simulink model "sysgenCORDICSinCos_mcode"  (Simulink 7.7)
settings: Solver=ode45  StartTime=0.0  StopTime=500  RelTol=1e-3
undefined symbols (not defined in the file or in its folder): Error_Measurement, sysgenCORDIC_lib
libraries: xbsIndex_r4 x23, dspobslib x9, dspstat3 x4, dspswit3 x2, xbsCopyrightNotice_r4 x1, simulink x1
settings Model: Creator=haibing  LastModifiedBy=douangp
settings DataIOCC: SignalLoggingName=sigsOut
settings OptimizationCC: InlineInvariantSignals=on  InitFltsAndDblsToZero=on
settings DebuggingCC: SaveWithParameterizedLinksMsg=none  SignalResolutionControl=TryResolveAllWithWarning  SolverPrmCheckMsg=none  MultiTaskDSMMsg=warning  MultiTaskCondExecSysMsg=none  StrictBusMsg=None
settings HardwareCC: TargetUnknown=on
settings RTWCC: IncludeERTFirstTime=on
settings GRTTargetCC: TargetFcnLib=ansi_tfl_tmw.mat

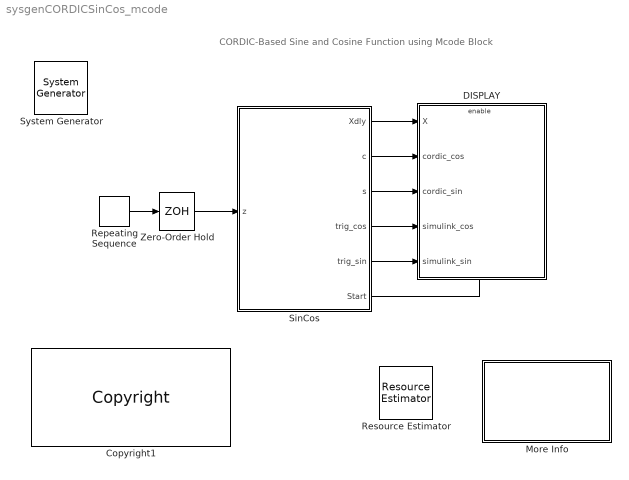
== system sysgenCORDICSinCos_mcode ==
  note: CORDIC-Based Sine and Cosine Function
      | using Mcode Block
  " System Generator" : xbsIndex_r4/ System Generator  Tag=genX  SystemSampleTime=-1  xilinxfamily=kintex7  part=xc7k325t  speed=-1  package=ffg900  synthesis_tool=XST  clock_wrapper=Clock Enables  directory=./sysgenCORDICSinCos_mcode_work  proj_type=Project Navigator  Synth_file=XST Defaults  Impl_file=ISE Defaults  testbench=on  simulink_period=1  sysclk_period=5.1  dcm_input_clock_period=100  incr_netlist=off  trim_vbits=Everywhere in SubSystem  dbl_ovrd=According to Block Masks  core_generation=Not Needed - Already Generated  run_coregen=off  deprecated_control=off  eval_field=0  block_type=sysgen
      settings: block_version=9.2.00
  Copyright1 : xbsCopyrightNotice_r4/Copyright  copyrighttext="Copyright (c) 2011  by  Xilinx, Inc. All rights reserved.<br><br>This file contains proprietary, confidential information of Xilinx, Inc., is distributed under license from Xilinx, Inc., and may be used, copied and/or disclosed only pursuant to the terms of a valid license agreement with Xilinx, Inc. Xilinx hereby grants you a license to use this file solely for design, simulation, implementation and creation of design files limited to Xilinx devices or technologies. Use with non-Xilinx devices or technologies is expressly prohibited and immediately terminates your license unless covered by a separate agreement.<br><br>Xilinx is providing this design, code, or information \"as-is\" solely for use in developing programs and solutions for Xilinx devices, with no obligation on the part of Xilinx to provide support. By providing this design, code, or information as one possible implementation of this feature, application or standard, Xilinx is making no representation that this implementation is free from any claims of infringement. You are responsible for obtaining any rights you may require for your implementation. Xilinx expressly disclaims any warranty whatsoever with respect to the adequacy of the implementation, including but not limited to any warranties or representations that this implementation is free from claims of infringement, implied warranties of merchantability or fitness for a particular purpose.<br><br>Xilinx products are not intended for use in life support appliances, devices, or systems. Use in such applications is expressly prohibited.<br><br>Any modifications that are made to the Source Code are done at the user's sole risk and will be unsupported.<br><br>This copyright and support notice must be retained as part of this text at all times. (c) Copyright 1995-2011 Xilinx, Inc. All rights reserved."  block_type=copyright
      settings: block_version=10.1.00
      settings: infoedit=|
      | Copyright(C) 2008 by  Xilinx, Inc. All rights reserved.<br>
      | <br>
      | This file contains proprietary, confidential information of Xilinx, Inc., is distributed under license
      | from Xilinx, Inc., and may be used, copied and/or disclosed only pursuant to the terms of a valid license
      | agreement with Xilinx, Inc. Xilinx hereby grants you a license to use this file solely for design,
      | simulation, implementation and creation of design files limited to Xilinx devices or technologies. Use
      | with non-Xilinx devices or technologies is expressly prohibited and immediately terminates your license
      | unless covered by a separate agreement.<br>
      | <br>
      | Xilinx is providing this design, code, or information "as-is" solely for use in developing programs and
      | solutions for Xilinx devices, with no obligation on the part of Xilinx to provide support. By providing
      | this design, code, or information as one possible implementation of this feature, application or standard,
      | Xilinx is making no representation that this implementation is free from any claims of infringement. You
      | are responsible for obtaining any rights you may require for your implementation. Xilinx expressly disclaims
      | any warranty whatsoever with respect to the adequacy of the implementation, including but not limited to any
      | warranties or representations that this implementation is free from claims of infringement, implied warranties
      | of merchantability or fitness for a particular purpose.<br>
      | <br>
      | Xilinx products are not intended for use in life support appliances, devices, or systems. Use in such
      | applications is expressly prohibited.<br>
      | <br>
      | Any modifications that are made to the Source Code are done at the user's sole risk and will be unsupported.<br>
      | <br>
      | This copyright and support notice must be retained as part of this text at all times.
      | (c) Copyright 1995-2008 Xilinx, Inc. All rights reserved.
  DISPLAY : Subsystem  TreatAsAtomicUnit=on
  More Info : Subsystem
      mask Display: disp('Double click\n for\n more information.')
  Repeating Sequence : simulink/Sources/Repeating Sequence  SystemSampleTime=-1  rep_seq_t=0:1:201  rep_seq_y=-pi:1/32:pi
  Resource Estimator : xbsIndex_r4/Resource Estimator  Tag=resEstTag  Slices=324  FFs=532  BRAMs=0  LUTs=556  IOBs=48  EBMs=0  TBUFs=0  xl_use_estimator_area=off  est_options=Estimate  xl_estimator_area=[324 532 0 556 48 0 0]  mrp_directory=./sysgenCORDIC_work_test  simulink_period=1  block_type=resource_estimator
      settings: AttributesFormatString=Resource\nEstimator  block_version=9.2.00
  SinCos : Subsystem  mask{pe_stages=8, pe_nbits=16, pe_binpt=13}
      mask prompts: pe_stages "Stages"; pe_nbits "Data Width"; pe_binpt "Binary Point"
      mask init:
      | [bg,fg] = xlcmap('XBlock',0);
      | iPos = get_param(gcb,'Position');
      | iWidth=iPos(3)-iPos(1); iHeight=iPos(4)-iPos(2);
      | iCx=iWidth/2;
      | iCy=iHeight/2;
      | [logoX, logoY] = xlogo(iPos);
      | 
      | pipeline = ones(1, pe_stages);
      | 
      | stages = round(sum(abs(pe_stages)));
      | if (stages == 0)
      | 	stages = 1;
      | end
      | x = zeros(1,stages);
      | pipe_size = max(size(pipeline));
      | if pipe_size >= stages
      | 	x(1,1:stages) = pipeline(1,1:stages);
      | else
      | 	x(1,1:pipe_size) = pipeline(1,1:pipe_size);
      | end
      | 
      | cordic_pe = find_system(gcb, 'LookUnderMasks', 'all', 'FollowLinks','on','masktype', 'CORDIC parallel PE');
      | a = find_system(cordic_pe{1}, 'LookUnderMasks', 'all', 'FollowLinks','on','masktype', 'CORDIC iteration PE');
      | prev_stages = length(a);
      | 
      | find_system(bdroot(gcs), 'lookUnderMasks', 'all', 'FollowLinks','on');
      | 
      | if (stages ~=prev_stages)
      |   pipeline=x;
      |     
      |   for i= 2:length(a)
      |     for j=1:3
      | 	  delete_line(cordic_pe{1}, ['CORDIC PE' int2str(i-1) '/' int2str(j)], ['CORDIC PE' int2str(i) '/' int2str(j)]);
      |     end
      |   end
      |     if length(a)>0,
      |       delete_line(cordic_pe{1}, 'x/1', 'CORDIC PE1/1');
      |       delete_line(cordic_pe{1}, 'y/1', 'CORDIC PE1/2');
      |       delete_line(cordic_pe{1}, 'z/1', 'CORDIC PE1/3');
      |       delete_line(cordic_pe{1}, ['CORDIC PE' int2str(length(a)) '/1'],'X/1');
      |       delete_line(cordic_pe{1}, ['CORDIC PE' int2str(length(a)) '/2'],'Y/1');
      |       delete_line(cordic_pe{1}, ['CORDIC PE' int2str(length(a)) '/3'],'Terminator/1');
      |     elseif length(a)==0
      |       temp_port=get_param([cordic_pe{1} '/x'],'porthandles');
      |       temp_line=get_param(temp_port.Outport,'line');
      |       if temp_line>=0  delete_line(temp_line); end
      |       temp_port=get_param([cordic_pe{1} '/y'],'porthandles');
      |       temp_line=get_param(temp_port.Outport,'line');
      |       if temp_line>=0  delete_line(temp_line); end
      |       temp_port=get_param([cordic_pe{1} '/z'],'porthandles');
      |       temp_line=get_param(temp_port.Outport,'line');
      |       if temp_line>=0  delete_line(temp_line); end
      |     end
      | 
      |     for i=2:length(a)
      |       delete_block(a{i});
      |     end
      |     for i=2:stages,
      |         add_block([cordic_pe{1} '/CORDIC PE1'], [cordic_pe{1} '/CORDIC PE' int2str(i)], 'ii', int2str(i-1),'pe_nbits', 'pe_nbits','pe_binpt', 'pe_binpt','pipeline',['pipeline(1,' int2str(i) ')'],'position',[150+(i-1)*125, 70, 205+(i-1)*125, 130]);
      |     end
      | 
      |     for i= 2:stages,
      |       for j=1:3
      | 		add_line(cordic_pe{1}, ['CORDIC PE' int2str(i-1) '/' int2str(j)], ['CORDIC PE' int2str(i) '/' int2str(j)], 'autorouting', 'on');
      |       end
      |     end
      | 
      |     if stages==0
      |       add_line(cordic_pe{1}, 'x/1', 'X/1', 'autorouting', 'on');
      |       add_line(cordic_pe{1}, 'y/1', 'Terminator/1', 'autorouting', 'on');
      |       add_line(cordic_pe{1}, 'z/1', 'Z/1', 'autorouting', 'on');
      |     elseif stages>0
      |       add_line(cordic_pe{1}, 'x/1', 'CORDIC PE1/1', 'autorouting', 'on');
      |       add_line(cordic_pe{1}, 'y/1', 'CORDIC PE1/2', 'autorouting', 'on');
      |       add_line(cordic_pe{1}, 'z/1', 'CORDIC PE1/3', 'autorouting', 'on');
      | 
      |       set_param([cordic_pe{1} '/' 'X'], 'Position', [150+stages*125, 72, 180+stages*125, 86]);
      |       set_param([cordic_pe{1} '/' 'Y'], 'Position', [210+stages*125, 92, 225+stages*125, 108]);
      |       set_param([cordic_pe{1} '/' 'Terminator'], 'Position', [240+stages*125, 113, 270+stages*125, 127]);
      | 
      |       add_line(cordic_pe{1}, ['CORDIC PE' int2str(stages) '/1'], 'X/1', 'autorouting', 'on');
      |       add_line(cordic_pe{1}, ['CORDIC PE' int2str(stages) '/2'], 'Y/1', 'autorouting', 'on');
      |       add_line(cordic_pe{1}, ['CORDIC PE' int2str(stages) '/3'],'Terminator/1', 'autorouting', 'on');
      | 
      |       % force a "compile" of the constituent constant blocks to
      |       % workaround a data propagation problem
      |       find_system(cordic_pe{1}, 'LookUnderMasks', 'all', 'FollowLinks', 'on', 'MaskType','Xilinx Constant Block');
      |   end
      | end
      | latency = sum(x) + 5;
      | str = sprintf('-%d',latency);
      mask Display:
      | patch([0 iWidth iWidth 0],[0 0 iHeight iHeight] , bg);
      | patch(logoX,logoY , fg);
      | 
      | text(iCx-6,iCy,'z');
      | text(iCx,iCy+4,str);
      | 
      | port_label('input',1,'z');
      | port_label('output',1,'z_dly');
      | port_label('output',2,'cordic_cos');
      | port_label('output',3,'cordic_sin');
      | port_label('output',4,'simulink_cos');
      | port_label('output',5,'simulink_sin');
      | port_label('output',6,'Start');
      | plot([0 0 iWidth iWidth 0], [0 iHeight iHeight 0 0]);
  Zero-Order Hold : ZeroOrderHold
  wires:
  Repeating Sequence/1 -> Zero-Order Hold/1
  Zero-Order Hold/1 -> SinCos/1(z)
  SinCos/1(Xdly) -> DISPLAY/1(X)
  SinCos/2(c) -> DISPLAY/2(cordic_cos)
  SinCos/3(s) -> DISPLAY/3(cordic_sin)
  SinCos/4(trig_cos) -> DISPLAY/4(simulink_cos)
  SinCos/5(trig_sin) -> DISPLAY/5(simulink_sin)
  SinCos/6(Start) -> DISPLAY/Enable

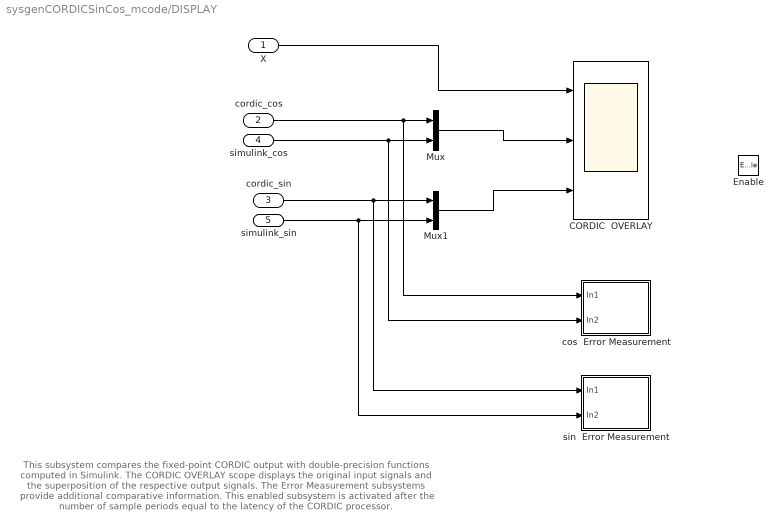
== system sysgenCORDICSinCos_mcode/DISPLAY ==
  note: This subsystem compares the fixed-point CORDIC output with double-precision functions computed in Simulink. The CORDIC OVERLAY scope
      | displays the original input signals and the superposition of the respective output signals.  The Error Measurement subsystems provide additional
      | comparative information.  This enabled subsystem is activated after the number of sample periods equal to the latency of the CORDIC processor.
  X : Inport
  cordic_cos : Inport  Port=2
  cordic_sin : Inport  Port=3
  simulink_cos : Inport  Port=4
  simulink_sin : Inport  Port=5
  Enable : EnablePort
  CORDIC  OVERLAY : Scope  NumInputPorts=3
      settings: TimeRange=500  YMin=-4~-1~-1.5  YMax=4~1.5~1.5
  Mux : Mux  Inputs=2
  Mux1 : Mux  Inputs=2
  cos  Error Measurement : Subsystem  AncestorBlock=sysgenCORDIC_lib/Error_Measurement
      mask Type: Error Measurement
  sin  Error Measurement : Subsystem
      mask Type: Error Measurement
  wires:
  Mux/1 -> CORDIC  OVERLAY/2
  Mux1/1 -> CORDIC  OVERLAY/3
  simulink_sin/1 -> sin  Error Measurement/2(In2), Mux1/2
  cordic_sin/1 -> sin  Error Measurement/1(In1), Mux1/1
  X/1 -> CORDIC  OVERLAY/1
  simulink_cos/1 -> cos  Error Measurement/2(In2), Mux/2
  cordic_cos/1 -> cos  Error Measurement/1(In1), Mux/1

== system sysgenCORDICSinCos_mcode/More Info ==
  note: CORDIC-Based Sine and Cosine Function using Mcode Block
  note: This design implements a fully parallel CORDIC  (COordinate Rotation DIgital Computer) algorithm in rotational mode that computes
      | the sine and cosine of the input angle z between +/- pi.
      |
      | The CORDIC algorithm is attractive for an FPGA implementation because it consists primarily of shift and add operations.
      | An N-bit adder/subtractor  requiries only N/2 logic slices.  The CORDIC subsystem is masked, and allows customization of bit precision,
      | the number of processing elements (PEs) in the CORDIC engine and the ability to pieline each individual stage.
      |
      |
      | References:
      | J. E. Volder, "The CORDIC Trigonometric Computing Technique", IRE Trans. On Electronic Computers, Vol. EC-8,  1959, pp. 330-334.
      | J. S. Walther, "A Unified Algorithm for Elementary Functions", Spring Joint Computer Conference (1971) pp. 379-385.
      | Yu Hen Hu, "CORDIC-Based VLSI Architectures for Digital Signal Processing", IEEE Signal Processing Magazine, pp. 17-34, July 1992.

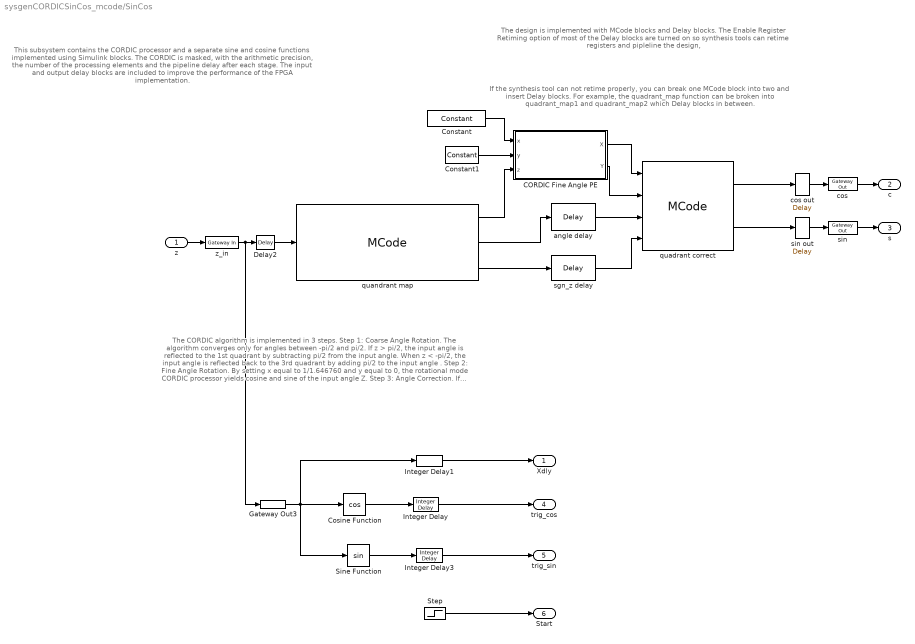
== system sysgenCORDICSinCos_mcode/SinCos ==
  note: This subsystem contains the CORDIC processor and a separate sine and cosine functions implemented using Simulink blocks.
      | The CORDIC is masked, with the arithmetic precision, the number of the processing elements and the pipeline delay after each
      | stage. The input and output delay blocks are included to improve the performance of the FPGA implementation.
  note: The CORDIC algorithm is implemented in 3 steps.
      |
      | Step 1: Coarse Angle Rotation.  The algorithm converges only for angles between -pi/2 and pi/2. If  z > pi/2, the input angle is reflected
      |  to the 1st quadrant by subtracting pi/2 from the input angle. When z < -pi/2, the input angle is reflected back to the 3rd quadrant by adding
      | pi/2 to the input angle .
      |
      | Step 2: Fine Angle Rotation.  By setting x equal to 1/1.646760 and y equal to 0, the rotational mode CORDIC processor yields cosine and sine
      | of the input angle Z.
      |
      | Step 3: Angle Correction. If there was a reflection applied in Step 1, this step applies the appropriate correction .
  note: If the synthesis tool can not retime properly, you can break one
      | MCode block into two and insert Delay blocks. For example,
      | the quadrant_map function can be broken into quadrant_map1
      | and quadrant_map2 which Delay blocks in between.
  note: The design is implemented with MCode blocks and Delay blocks.
      | The Enable Register Retiming option of most of the Delay blocks
      | are turned on so synthesis tools can retime registers and
      | pipleline the design,
  z : Inport
  CORDIC Fine Angle PE : Subsystem  mask(CORDIC parallel PE){}
      mask init:
      | [bg,fg] = xlcmap('XBlock',0);
      | iPos = get_param(gcb,'Position');
      | iWidth=iPos(3)-iPos(1); iHeight=iPos(4)-iPos(2);
      | iCx=iWidth/2;
      | iCy=iHeight/2;
      | [logoX, logoY] = xlogo(iPos);
      mask Display:
      | patch([0 iWidth iWidth 0],[0 0 iHeight iHeight] , bg);
      | patch(logoX,logoY , fg);
      | port_label('input',1,'x');
      | port_label('input',2,'y');
      | port_label('input',3,'z');
      | port_label('output',1,'X');
      | port_label('output',2,'Y');
      | plot([0 0 iWidth iWidth 0], [0 iHeight iHeight 0 0]);
  Constant : xbsIndex_r4/Constant  const=1/1.646760  gui_display_data_type=Fixed-point  arith_type=Unsigned  n_bits=pe_nbits  bin_pt=pe_binpt  preci_type=Single  exp_width=8  frac_width=24  explicit_period=on  period=1  equ=P=C  opselect=C  inp2=PCIN>>17  opr=+  inp1=P  carry=CIN  dbl_ovrd=off  block_type=constant
      settings: block_version=VER_STRING_GOES_HERE
  Constant1 : xbsIndex_r4/Constant  const=0  gui_display_data_type=Fixed-point  arith_type=Unsigned  n_bits=pe_nbits  bin_pt=pe_binpt  preci_type=Single  exp_width=8  frac_width=24  explicit_period=on  period=1  equ=P=C  opselect=C  inp2=PCIN>>17  opr=+  inp1=P  carry=CIN  dbl_ovrd=off  block_type=constant
      settings: block_version=VER_STRING_GOES_HERE
  Cosine Function : Trigonometry  Operator=cos
  Delay2 : xbsIndex_r4/Delay  rst=off  infoeditControl=Selection of Reset will increase slice count due to use of real FFs and instead of SRLs  en=off  latency=1  dbl_ovrd=off  reg_retiming=off  block_type=delay
      settings: infoedit="Delay line having  configurable length.<P><P>Hardware notes: A delay line is a chain, each link of which is an SRL16 followed by a flip-flop. If register retiming is enabled, the delay line is a chain of flip-flops."  xl_area=[8 16 0 0 0 0 0]  block_version=VER_STRING_GOES_HERE
  Gateway Out3 : xbsIndex_r4/Gateway Out  hdl_port=off  timing_constraint=None  locs_specified=off  LOCs={}  block_type=gatewayout
      settings: infoedit="Gateway out block.  Converts Xilinx fixed point inputs into ouputs of type Simulink integer, double, or fixed point.<P><P>Hardware notes:  In hardware these blocks become top level output ports or are discarded, depending on how they are configured."  xl_area=[0 0 0 0 0 0 0]  block_version=VER_STRING_GOES_HERE
  Integer Delay : dspobslib/Integer Delay  delay=latency  ic=0  reset_popup=None
  Integer Delay1 : dspobslib/Integer Delay  delay=latency  ic=0  reset_popup=None
  Integer Delay3 : dspobslib/Integer Delay  delay=latency  ic=0  reset_popup=None
  Sine Function : Trigonometry
  Step : Step  Time=latency  SampleTime=1
  angle delay : xbsIndex_r4/Delay  rst=off  infoeditControl=Selection of Reset will increase slice count due to use of real FFs and instead of SRLs  en=off  latency=sum(pipeline)  dbl_ovrd=off  reg_retiming=off  block_type=delay
      settings: infoedit="Delay line having  configurable length.<P><P>Hardware notes: A delay line is a chain, each link of which is an SRL16 followed by a flip-flop. If register retiming is enabled, the delay line is a chain of flip-flops."  xl_area=[0, 0, 0, 0, 0, 0, 0]  block_version=VER_STRING_GOES_HERE
  cos : xbsIndex_r4/Gateway Out  hdl_port=on  timing_constraint="Data Rate;  Set 'FAST' Attribute"  locs_specified=off  LOCs={}  block_type=gatewayout
      settings: infoedit="Gateway out block.  Converts Xilinx fixed point inputs into ouputs of type Simulink integer, double, or fixed point.<P><P>Hardware notes:  In hardware these blocks become top level output ports or are discarded, depending on how they are configured."  xl_area=[0 0 0 0 16 0 0]  block_version=VER_STRING_GOES_HERE
  cos out : xbsIndex_r4/Delay  rst=off  infoeditControl=Selection of Reset will increase slice count due to use of real FFs and instead of SRLs  en=off  latency=1  dbl_ovrd=off  reg_retiming=off  block_type=delay
      settings: infoedit="Delay line having  configurable length.<P><P>Hardware notes: A delay line is a chain, each link of which is an SRL16 followed by a flip-flop. If register retiming is enabled, the delay line is a chain of flip-flops."  xl_area=[0, 0, 0, 0, 0, 0, 0]  block_version=VER_STRING_GOES_HERE
  quadrant correct : xbsIndex_r4/MCode  mfname=quadrant_correct_lat  explicit_period=off  period=1  dbl_ovrd=off  enable_stdout=off  enable_debug=off  suppress_output=off  defparams={'nbits', pe_nbits,'binpt', pe_binpt,'lat',1}  hide_port_list={}  block_type=mcode
      settings: xl_area=[0, 0, 0, 0, 0, 0, 0]  block_version=8.1
  quandrant map : xbsIndex_r4/MCode  mfname=quadrant_map_lat2  explicit_period=off  period=1  dbl_ovrd=off  enable_stdout=off  enable_debug=off  suppress_output=off  defparams={'nbits', pe_nbits,'binpt', pe_binpt,'lat',2}  hide_port_list={}  block_type=mcode
      settings: xl_area=[0, 0, 0, 0, 0, 0, 0]  block_version=8.1
  sgn_z delay : xbsIndex_r4/Delay  rst=off  infoeditControl=Selection of Reset will increase slice count due to use of real FFs and instead of SRLs  en=off  latency=sum(pipeline)  dbl_ovrd=off  reg_retiming=off  block_type=delay
      settings: infoedit="Delay line having  configurable length.<P><P>Hardware notes: A delay line is a chain, each link of which is an SRL16 followed by a flip-flop. If register retiming is enabled, the delay line is a chain of flip-flops."  xl_area=[0, 0, 0, 0, 0, 0, 0]  block_version=VER_STRING_GOES_HERE
  sin : xbsIndex_r4/Gateway Out  hdl_port=on  timing_constraint="Data Rate;  Set 'FAST' Attribute"  locs_specified=off  LOCs={}  block_type=gatewayout
      settings: infoedit="Gateway out block.  Converts Xilinx fixed point inputs into ouputs of type Simulink integer, double, or fixed point.<P><P>Hardware notes:  In hardware these blocks become top level output ports or are discarded, depending on how they are configured."  xl_area=[0 0 0 0 16 0 0]  block_version=VER_STRING_GOES_HERE
  sin out : xbsIndex_r4/Delay  rst=off  infoeditControl=Selection of Reset will increase slice count due to use of real FFs and instead of SRLs  en=off  latency=1  dbl_ovrd=off  reg_retiming=off  block_type=delay
      settings: infoedit="Delay line having  configurable length.<P><P>Hardware notes: A delay line is a chain, each link of which is an SRL16 followed by a flip-flop. If register retiming is enabled, the delay line is a chain of flip-flops."  xl_area=[0, 0, 0, 0, 0, 0, 0]  block_version=VER_STRING_GOES_HERE
  z_in : xbsIndex_r4/Gateway In  gui_display_data_type=Fixed-point  arith_type="Signed  (2's comp)"  n_bits=pe_nbits  bin_pt=pe_binpt  preci_type=Single  exp_width=8  frac_width=24  quantization="Round  (unbiased: +/- Inf)"  overflow=Saturate  period=1  dbl_ovrd=off  timing_constraint=None  locs_specified=off  LOCs={}  hdl_port=on  block_type=gatewayin
      settings: infoedit="Gateway in block.  Converts inputs of type Simulink integer, double and fixed point to  Xilinx fixed point type.<P><P>Hardware notes:  In hardware these blocks become top level input ports."  xl_area=[0 0 0 0 16 0 0]  block_version=VER_STRING_GOES_HERE
  Xdly : Outport
  c : Outport  Port=2
  s : Outport  Port=3
  trig_cos : Outport  Port=4
  trig_sin : Outport  Port=5
  Start : Outport  Port=6
  wires:
  z_in/1 -> Delay2/1, Gateway Out3/1
  quandrant map/1 -> CORDIC Fine Angle PE/3(z)
  CORDIC Fine Angle PE/1(X) -> quadrant correct/1
  CORDIC Fine Angle PE/2(Y) -> quadrant correct/2
  angle delay/1 -> quadrant correct/3
  sgn_z delay/1 -> quadrant correct/4
  Constant/1 -> CORDIC Fine Angle PE/1(x)
  Constant1/1 -> CORDIC Fine Angle PE/2(y)
  Delay2/1 -> quandrant map/1
  z/1 -> z_in/1
  cos out/1 -> cos/1
  sin out/1 -> sin/1
  Gateway Out3/1 -> Integer Delay1/1, Sine Function/1, Cosine Function/1
  Step/1 -> Start/1
  Integer Delay3/1 -> trig_sin/1
  Integer Delay/1 -> trig_cos/1
  Sine Function/1 -> Integer Delay3/1
  Integer Delay1/1 -> Xdly/1
  Cosine Function/1 -> Integer Delay/1
  cos/1 -> c/1
  sin/1 -> s/1
  quandrant map/2 -> angle delay/1
  quandrant map/3 -> sgn_z delay/1
  quadrant correct/1 -> cos out/1
  quadrant correct/2 -> sin out/1

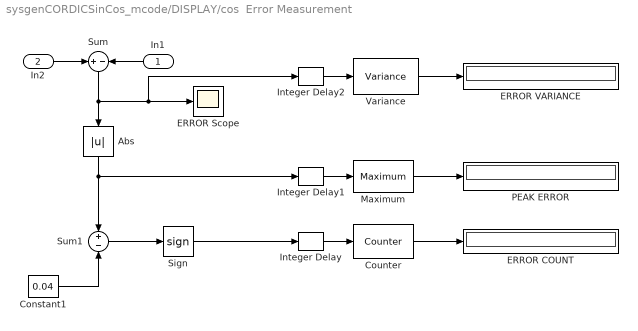
== system sysgenCORDICSinCos_mcode/DISPLAY/cos  Error Measurement ==
  In1 : Inport
  In2 : Inport  Port=2
  Abs : Abs  SaturateOnIntegerOverflow=on
  Constant1 : Constant  Value=0.04
  Counter : dspswit3/Counter  Direction=Up  CountEvent=Rising edge  CounterSize=User defined  MaxCount=200000000  InitialCount=0  Output=Count  HitValue=32  ResetInput=off  SamplesPerFrame=1  Ts=1  CntDtype=double  HitDtype=Logical
  ERROR Scope : Scope
      settings: TimeRange=10000  YMin=-0.0006  YMax=0.0005  SaveName=ScopeData2
  ERROR COUNT : Display
      settings: Format=long_e
  ERROR VARIANCE : Display
      settings: Format=long_e
  Integer Delay : dspobslib/Integer Delay  delay=1  ic=0  reset_popup=None
  Integer Delay1 : dspobslib/Integer Delay  delay=1  ic=0  reset_popup=None
  Integer Delay2 : dspobslib/Integer Delay  delay=1  ic=0  reset_popup=None
  Maximum : dspstat3/Maximum  fcn=Running  reset=None  InputProcessing=Inherited (this choice will be removed - see release notes)  indexBase=One  operateOver=Each column  Dimension=1  colComp=on  operation=maximum  roiEnable=off  roiType=Rectangles  roiPortion=Entire ROI  roiOutput=Individual statistics for each ROI  roiFlag=off  accumDataTypeStr=Inherit: Same as product output  accumLastDataTypeStr=Inherit: Same as product output  roundingMode=Floor  overflowMode=off
  PEAK ERROR : Display
      settings: Format=long_e
  Sign : Signum
  Sum : Sum  Inputs=+-  SaturateOnIntegerOverflow=on  InputSameDT=on  OutDataTypeStr=Inherit: Same as first input
  Sum1 : Sum  Inputs=+-  SaturateOnIntegerOverflow=on  InputSameDT=on  OutDataTypeStr=Inherit: Same as first input
  Variance : dspstat3/Variance  run=on  reset_popup=None  InputProcessing=Inherited (this choice will be removed - see release notes)  directionMode=Each column  dimension=1  treatSBRowAsCol=on  roiEnable=off  roiType=Rectangles  roiPortion=Entire ROI  roiOutput=Individual statistics for each ROI  roiFlag=off  roundingMode=Floor  overflowMode=off
  wires:
  In2/1 -> Sum/1
  In1/1 -> Sum/2
  Integer Delay2/1 -> Variance/1
  Integer Delay1/1 -> Maximum/1
  Integer Delay/1 -> Counter/1
  Maximum/1 -> PEAK ERROR/1
  Variance/1 -> ERROR VARIANCE/1
  Counter/1 -> ERROR COUNT/1
  Sign/1 -> Integer Delay/1
  Sum1/1 -> Sign/1
  Abs/1 -> Integer Delay1/1, Sum1/1
  Constant1/1 -> Sum1/2
  Sum/1 -> Integer Delay2/1, ERROR Scope/1, Abs/1

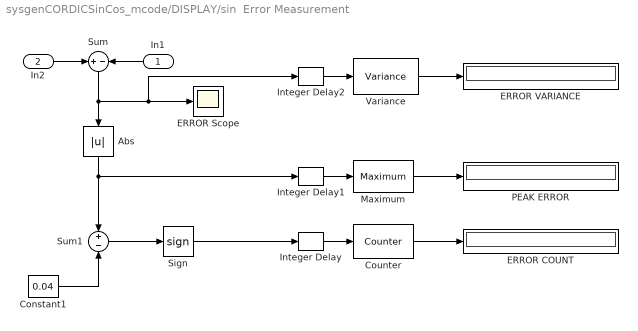
== system sysgenCORDICSinCos_mcode/DISPLAY/sin  Error Measurement ==
  In1 : Inport
  In2 : Inport  Port=2
  Abs : Abs  SaturateOnIntegerOverflow=on
  Constant1 : Constant  Value=0.04
  Counter : dspswit3/Counter  Direction=Up  CountEvent=Rising edge  CounterSize=User defined  MaxCount=200000000  InitialCount=0  Output=Count  HitValue=32  ResetInput=off  SamplesPerFrame=1  Ts=1  CntDtype=double  HitDtype=Logical
  ERROR Scope : Scope
      settings: TimeRange=10000  YMin=-0.0006  YMax=0.0005  SaveName=ScopeData2
  ERROR COUNT : Display
      settings: Format=long_e
  ERROR VARIANCE : Display
      settings: Format=long_e
  Integer Delay : dspobslib/Integer Delay  delay=1  ic=0  reset_popup=None
  Integer Delay1 : dspobslib/Integer Delay  delay=1  ic=0  reset_popup=None
  Integer Delay2 : dspobslib/Integer Delay  delay=1  ic=0  reset_popup=None
  Maximum : dspstat3/Maximum  fcn=Running  reset=None  InputProcessing=Inherited (this choice will be removed - see release notes)  indexBase=One  operateOver=Each column  Dimension=1  colComp=on  operation=maximum  roiEnable=off  roiType=Rectangles  roiPortion=Entire ROI  roiOutput=Individual statistics for each ROI  roiFlag=off  accumDataTypeStr=Inherit: Same as product output  accumLastDataTypeStr=Inherit: Same as product output  roundingMode=Floor  overflowMode=off
  PEAK ERROR : Display
      settings: Format=long_e
  Sign : Signum
  Sum : Sum  Inputs=+-  SaturateOnIntegerOverflow=on  InputSameDT=on  OutDataTypeStr=Inherit: Same as first input
  Sum1 : Sum  Inputs=+-  SaturateOnIntegerOverflow=on  InputSameDT=on  OutDataTypeStr=Inherit: Same as first input
  Variance : dspstat3/Variance  run=on  reset_popup=None  InputProcessing=Inherited (this choice will be removed - see release notes)  directionMode=Each column  dimension=1  treatSBRowAsCol=on  roiEnable=off  roiType=Rectangles  roiPortion=Entire ROI  roiOutput=Individual statistics for each ROI  roiFlag=off  roundingMode=Floor  overflowMode=off
  wires:
  In2/1 -> Sum/1
  In1/1 -> Sum/2
  Integer Delay2/1 -> Variance/1
  Integer Delay1/1 -> Maximum/1
  Integer Delay/1 -> Counter/1
  Maximum/1 -> PEAK ERROR/1
  Variance/1 -> ERROR VARIANCE/1
  Counter/1 -> ERROR COUNT/1
  Sign/1 -> Integer Delay/1
  Sum1/1 -> Sign/1
  Abs/1 -> Integer Delay1/1, Sum1/1
  Constant1/1 -> Sum1/2
  Sum/1 -> Integer Delay2/1, ERROR Scope/1, Abs/1

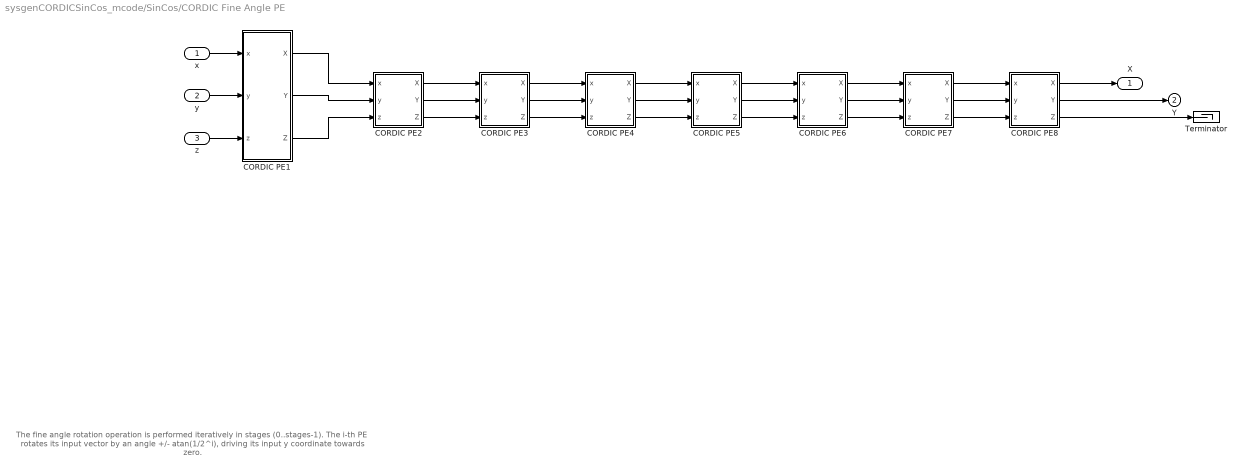
== system sysgenCORDICSinCos_mcode/SinCos/CORDIC Fine Angle PE ==
  note: The fine angle rotation operation is performed iteratively in stages (0..stages-1).
      | The i-th PE rotates its input vector by an angle +/- atan(1/2^i), driving its input y coordinate towards zero.
  x : Inport
  y : Inport  Port=2
  z : Inport  Port=3
  CORDIC PE1 : Subsystem  mask(CORDIC iteration PE){ii=0, pe_nbits=pe_nbits, pe_binpt=pe_binpt, epsilon_k_fcn=atan, epsilon_k=, pipeline=pipeline(1,1)}
      mask prompts: ii "Iteration Index ii"; pe_nbits "Number of X,Y,Z Bits"; pe_binpt "X,Y,Z Binary Point Position"; epsilon_k_fcn "Epsilon_k Function"; pipeline "Pipeline Latency"
      mask init:
      | [bg,fg] = xlcmap('XBlock',0);
      | iPos = get_param(gcb,'Position');
      | iWidth=iPos(3)-iPos(1); iHeight=iPos(4)-iPos(2);
      | iCx=iWidth/2;
      | iCy=iHeight/2;
      | [logoX, logoY] = xlogo(iPos);
      | 
      | set_param(gcb, 'LinkStatus', 'none');
      | switch epsilon_k_fcn
      |   case 1
      |     epsilon_k = atan(1/2^ii);
      |   case 2
      |     epsilon_k = atanh(1/2^ii);
      | end
      mask StyleString: edit,edit,edit,popup(atan|atanh),edit,edit
      mask Display:
      | patch([0 iWidth iWidth 0],[0 0 iHeight iHeight] , bg);
      | patch(logoX,logoY , fg);
      | port_label('input',1,'x');
      | port_label('input',2,'y');
      | port_label('input',3,'z');
      | 
      | port_label('output',1,'X');
      | port_label('output',2,'Y');
      | port_label('output',3,'Z');
      | plot([0 0 iWidth iWidth 0], [0 iHeight iHeight 0 0]);
  CORDIC PE2 : Subsystem  mask(CORDIC iteration PE){ii=1, pe_nbits=pe_nbits, pe_binpt=pe_binpt, epsilon_k_fcn=atan, epsilon_k=, pipeline=pipeline(1,2)}
      mask prompts: ii "Iteration Index ii"; pe_nbits "Number of X,Y,Z Bits"; pe_binpt "X,Y,Z Binary Point Position"; epsilon_k_fcn "Epsilon_k Function"; pipeline "Pipeline Latency"
      mask init: same as sysgenCORDICSinCos_mcode/SinCos/CORDIC Fine Angle PE/CORDIC PE1
      mask StyleString: edit,edit,edit,popup(atan|atanh),edit,edit
      mask Display:
      | patch([0 iWidth iWidth 0],[0 0 iHeight iHeight] , bg);
      | patch(logoX,logoY , fg);
      | port_label('input',1,'x');
      | port_label('input',2,'y');
      | port_label('input',3,'z');
      | 
      | port_label('output',1,'X');
      | port_label('output',2,'Y');
      | port_label('output',3,'Z');
      | plot([0 0 iWidth iWidth 0], [0 iHeight iHeight 0 0]);
  CORDIC PE3 : Subsystem  mask(CORDIC iteration PE){ii=2, pe_nbits=pe_nbits, pe_binpt=pe_binpt, epsilon_k_fcn=atan, epsilon_k=, pipeline=pipeline(1,3)}
      mask prompts: ii "Iteration Index ii"; pe_nbits "Number of X,Y,Z Bits"; pe_binpt "X,Y,Z Binary Point Position"; epsilon_k_fcn "Epsilon_k Function"; pipeline "Pipeline Latency"
      mask init: same as sysgenCORDICSinCos_mcode/SinCos/CORDIC Fine Angle PE/CORDIC PE1
      mask StyleString: edit,edit,edit,popup(atan|atanh),edit,edit
      mask Display:
      | patch([0 iWidth iWidth 0],[0 0 iHeight iHeight] , bg);
      | patch(logoX,logoY , fg);
      | port_label('input',1,'x');
      | port_label('input',2,'y');
      | port_label('input',3,'z');
      | 
      | port_label('output',1,'X');
      | port_label('output',2,'Y');
      | port_label('output',3,'Z');
      | plot([0 0 iWidth iWidth 0], [0 iHeight iHeight 0 0]);
  CORDIC PE4 : Subsystem  mask(CORDIC iteration PE){ii=3, pe_nbits=pe_nbits, pe_binpt=pe_binpt, epsilon_k_fcn=atan, epsilon_k=, pipeline=pipeline(1,4)}
      mask prompts: ii "Iteration Index ii"; pe_nbits "Number of X,Y,Z Bits"; pe_binpt "X,Y,Z Binary Point Position"; epsilon_k_fcn "Epsilon_k Function"; pipeline "Pipeline Latency"
      mask init: same as sysgenCORDICSinCos_mcode/SinCos/CORDIC Fine Angle PE/CORDIC PE1
      mask StyleString: edit,edit,edit,popup(atan|atanh),edit,edit
      mask Display:
      | patch([0 iWidth iWidth 0],[0 0 iHeight iHeight] , bg);
      | patch(logoX,logoY , fg);
      | port_label('input',1,'x');
      | port_label('input',2,'y');
      | port_label('input',3,'z');
      | 
      | port_label('output',1,'X');
      | port_label('output',2,'Y');
      | port_label('output',3,'Z');
      | plot([0 0 iWidth iWidth 0], [0 iHeight iHeight 0 0]);
  CORDIC PE5 : Subsystem  mask(CORDIC iteration PE){ii=4, pe_nbits=pe_nbits, pe_binpt=pe_binpt, epsilon_k_fcn=atan, epsilon_k=, pipeline=pipeline(1,5)}
      mask prompts: ii "Iteration Index ii"; pe_nbits "Number of X,Y,Z Bits"; pe_binpt "X,Y,Z Binary Point Position"; epsilon_k_fcn "Epsilon_k Function"; pipeline "Pipeline Latency"
      mask init: same as sysgenCORDICSinCos_mcode/SinCos/CORDIC Fine Angle PE/CORDIC PE1
      mask StyleString: edit,edit,edit,popup(atan|atanh),edit,edit
      mask Display:
      | patch([0 iWidth iWidth 0],[0 0 iHeight iHeight] , bg);
      | patch(logoX,logoY , fg);
      | port_label('input',1,'x');
      | port_label('input',2,'y');
      | port_label('input',3,'z');
      | 
      | port_label('output',1,'X');
      | port_label('output',2,'Y');
      | port_label('output',3,'Z');
      | plot([0 0 iWidth iWidth 0], [0 iHeight iHeight 0 0]);
  CORDIC PE6 : Subsystem  mask(CORDIC iteration PE){ii=5, pe_nbits=pe_nbits, pe_binpt=pe_binpt, epsilon_k_fcn=atan, epsilon_k=, pipeline=pipeline(1,6)}
      mask prompts: ii "Iteration Index ii"; pe_nbits "Number of X,Y,Z Bits"; pe_binpt "X,Y,Z Binary Point Position"; epsilon_k_fcn "Epsilon_k Function"; pipeline "Pipeline Latency"
      mask init: same as sysgenCORDICSinCos_mcode/SinCos/CORDIC Fine Angle PE/CORDIC PE1
      mask StyleString: edit,edit,edit,popup(atan|atanh),edit,edit
      mask Display:
      | patch([0 iWidth iWidth 0],[0 0 iHeight iHeight] , bg);
      | patch(logoX,logoY , fg);
      | port_label('input',1,'x');
      | port_label('input',2,'y');
      | port_label('input',3,'z');
      | 
      | port_label('output',1,'X');
      | port_label('output',2,'Y');
      | port_label('output',3,'Z');
      | plot([0 0 iWidth iWidth 0], [0 iHeight iHeight 0 0]);
  CORDIC PE7 : Subsystem  mask(CORDIC iteration PE){ii=6, pe_nbits=pe_nbits, pe_binpt=pe_binpt, epsilon_k_fcn=atan, epsilon_k=, pipeline=pipeline(1,7)}
      mask prompts: ii "Iteration Index ii"; pe_nbits "Number of X,Y,Z Bits"; pe_binpt "X,Y,Z Binary Point Position"; epsilon_k_fcn "Epsilon_k Function"; pipeline "Pipeline Latency"
      mask init: same as sysgenCORDICSinCos_mcode/SinCos/CORDIC Fine Angle PE/CORDIC PE1
      mask StyleString: edit,edit,edit,popup(atan|atanh),edit,edit
      mask Display:
      | patch([0 iWidth iWidth 0],[0 0 iHeight iHeight] , bg);
      | patch(logoX,logoY , fg);
      | port_label('input',1,'x');
      | port_label('input',2,'y');
      | port_label('input',3,'z');
      | 
      | port_label('output',1,'X');
      | port_label('output',2,'Y');
      | port_label('output',3,'Z');
      | plot([0 0 iWidth iWidth 0], [0 iHeight iHeight 0 0]);
  CORDIC PE8 : Subsystem  mask(CORDIC iteration PE){ii=7, pe_nbits=pe_nbits, pe_binpt=pe_binpt, epsilon_k_fcn=atan, epsilon_k=, pipeline=pipeline(1,8)}
      mask prompts: ii "Iteration Index ii"; pe_nbits "Number of X,Y,Z Bits"; pe_binpt "X,Y,Z Binary Point Position"; epsilon_k_fcn "Epsilon_k Function"; pipeline "Pipeline Latency"
      mask init: same as sysgenCORDICSinCos_mcode/SinCos/CORDIC Fine Angle PE/CORDIC PE1
      mask StyleString: edit,edit,edit,popup(atan|atanh),edit,edit
      mask Display:
      | patch([0 iWidth iWidth 0],[0 0 iHeight iHeight] , bg);
      | patch(logoX,logoY , fg);
      | port_label('input',1,'x');
      | port_label('input',2,'y');
      | port_label('input',3,'z');
      | 
      | port_label('output',1,'X');
      | port_label('output',2,'Y');
      | port_label('output',3,'Z');
      | plot([0 0 iWidth iWidth 0], [0 iHeight iHeight 0 0]);
  Terminator : Terminator
  X : Outport
  Y : Outport  Port=2
  wires:
  CORDIC PE1/1(X) -> CORDIC PE2/1(x)
  CORDIC PE1/2(Y) -> CORDIC PE2/2(y)
  CORDIC PE1/3(Z) -> CORDIC PE2/3(z)
  CORDIC PE2/1(X) -> CORDIC PE3/1(x)
  CORDIC PE2/2(Y) -> CORDIC PE3/2(y)
  CORDIC PE2/3(Z) -> CORDIC PE3/3(z)
  CORDIC PE3/1(X) -> CORDIC PE4/1(x)
  CORDIC PE3/2(Y) -> CORDIC PE4/2(y)
  CORDIC PE3/3(Z) -> CORDIC PE4/3(z)
  CORDIC PE4/1(X) -> CORDIC PE5/1(x)
  CORDIC PE4/2(Y) -> CORDIC PE5/2(y)
  CORDIC PE4/3(Z) -> CORDIC PE5/3(z)
  CORDIC PE5/1(X) -> CORDIC PE6/1(x)
  CORDIC PE5/2(Y) -> CORDIC PE6/2(y)
  CORDIC PE5/3(Z) -> CORDIC PE6/3(z)
  CORDIC PE6/1(X) -> CORDIC PE7/1(x)
  CORDIC PE6/2(Y) -> CORDIC PE7/2(y)
  CORDIC PE6/3(Z) -> CORDIC PE7/3(z)
  CORDIC PE7/1(X) -> CORDIC PE8/1(x)
  CORDIC PE7/2(Y) -> CORDIC PE8/2(y)
  CORDIC PE7/3(Z) -> CORDIC PE8/3(z)
  x/1 -> CORDIC PE1/1(x)
  y/1 -> CORDIC PE1/2(y)
  z/1 -> CORDIC PE1/3(z)
  CORDIC PE8/1(X) -> X/1
  CORDIC PE8/2(Y) -> Y/1
  CORDIC PE8/3(Z) -> Terminator/1

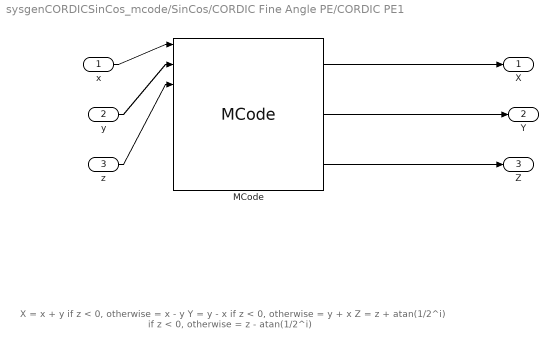
== system sysgenCORDICSinCos_mcode/SinCos/CORDIC Fine Angle PE/CORDIC PE1 ==
  note: X = x + y if z < 0, otherwise
      |    = x - y
      | Y = y - x if z < 0, otherwise
      |    = y + x
      | Z = z + atan(1/2^i) if z < 0, otherwise
      |    = z - atan(1/2^i)
  x : Inport
  y : Inport  Port=2
  z : Inport  Port=3
  MCode : xbsIndex_r4/MCode  mfname=cordic_pe_lat1  explicit_period=off  period=1  dbl_ovrd=off  enable_stdout=off  enable_debug=off  suppress_output=off  defparams={'shbits',ii,'epsilon', epsilon_k,'nbits', pe_nbits,'binpt', pe_binpt,'lat',pipeline}  hide_port_list={}  block_type=mcode
      settings: xl_area=[0, 0, 0, 0, 0, 0, 0]  block_version=8.1
  X : Outport
  Y : Outport  Port=2
  Z : Outport  Port=3
  wires:
  x/1 -> MCode/1
  y/1 -> MCode/2
  z/1 -> MCode/3
  MCode/1 -> X/1
  MCode/2 -> Y/1
  MCode/3 -> Z/1

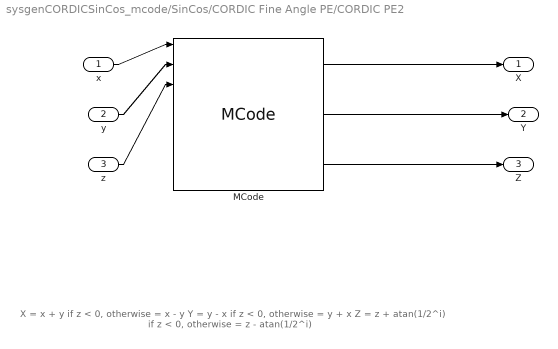
== system sysgenCORDICSinCos_mcode/SinCos/CORDIC Fine Angle PE/CORDIC PE2 ==
  note: X = x + y if z < 0, otherwise
      |    = x - y
      | Y = y - x if z < 0, otherwise
      |    = y + x
      | Z = z + atan(1/2^i) if z < 0, otherwise
      |    = z - atan(1/2^i)
  x : Inport
  y : Inport  Port=2
  z : Inport  Port=3
  MCode : xbsIndex_r4/MCode  mfname=cordic_pe_lat1  explicit_period=off  period=1  dbl_ovrd=off  enable_stdout=off  enable_debug=off  suppress_output=off  defparams={'shbits',ii,'epsilon', epsilon_k,'nbits', pe_nbits,'binpt', pe_binpt,'lat',pipeline}  hide_port_list={}  block_type=mcode
      settings: xl_area=[0, 0, 0, 0, 0, 0, 0]  block_version=8.1
  X : Outport
  Y : Outport  Port=2
  Z : Outport  Port=3
  wires:
  MCode/3 -> Z/1
  MCode/2 -> Y/1
  MCode/1 -> X/1
  z/1 -> MCode/3
  y/1 -> MCode/2
  x/1 -> MCode/1

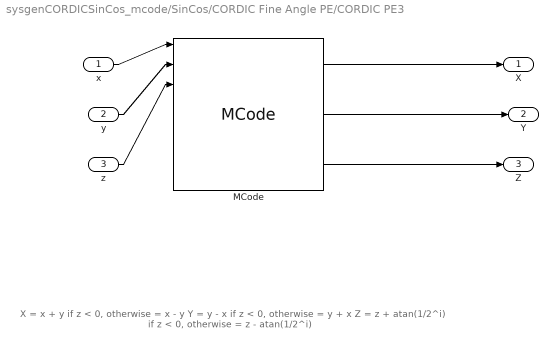
== system sysgenCORDICSinCos_mcode/SinCos/CORDIC Fine Angle PE/CORDIC PE3 ==
  note: X = x + y if z < 0, otherwise
      |    = x - y
      | Y = y - x if z < 0, otherwise
      |    = y + x
      | Z = z + atan(1/2^i) if z < 0, otherwise
      |    = z - atan(1/2^i)
  x : Inport
  y : Inport  Port=2
  z : Inport  Port=3
  MCode : xbsIndex_r4/MCode  mfname=cordic_pe_lat1  explicit_period=off  period=1  dbl_ovrd=off  enable_stdout=off  enable_debug=off  suppress_output=off  defparams={'shbits',ii,'epsilon', epsilon_k,'nbits', pe_nbits,'binpt', pe_binpt,'lat',pipeline}  hide_port_list={}  block_type=mcode
      settings: xl_area=[0, 0, 0, 0, 0, 0, 0]  block_version=8.1
  X : Outport
  Y : Outport  Port=2
  Z : Outport  Port=3
  wires:
  MCode/3 -> Z/1
  MCode/2 -> Y/1
  MCode/1 -> X/1
  z/1 -> MCode/3
  y/1 -> MCode/2
  x/1 -> MCode/1

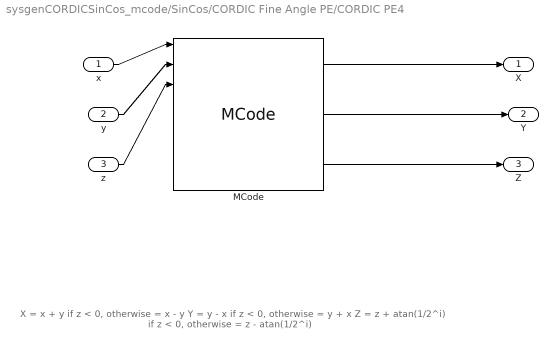
== system sysgenCORDICSinCos_mcode/SinCos/CORDIC Fine Angle PE/CORDIC PE4 ==
  note: X = x + y if z < 0, otherwise
      |    = x - y
      | Y = y - x if z < 0, otherwise
      |    = y + x
      | Z = z + atan(1/2^i) if z < 0, otherwise
      |    = z - atan(1/2^i)
  x : Inport
  y : Inport  Port=2
  z : Inport  Port=3
  MCode : xbsIndex_r4/MCode  mfname=cordic_pe_lat1  explicit_period=off  period=1  dbl_ovrd=off  enable_stdout=off  enable_debug=off  suppress_output=off  defparams={'shbits',ii,'epsilon', epsilon_k,'nbits', pe_nbits,'binpt', pe_binpt,'lat',pipeline}  hide_port_list={}  block_type=mcode
      settings: xl_area=[0, 0, 0, 0, 0, 0, 0]  block_version=8.1
  X : Outport
  Y : Outport  Port=2
  Z : Outport  Port=3
  wires:
  MCode/3 -> Z/1
  MCode/2 -> Y/1
  MCode/1 -> X/1
  z/1 -> MCode/3
  y/1 -> MCode/2
  x/1 -> MCode/1

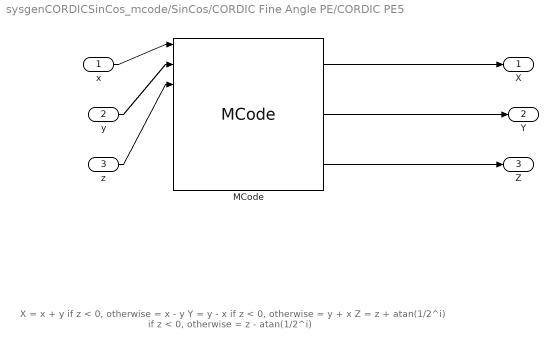
== system sysgenCORDICSinCos_mcode/SinCos/CORDIC Fine Angle PE/CORDIC PE5 ==
  note: X = x + y if z < 0, otherwise
      |    = x - y
      | Y = y - x if z < 0, otherwise
      |    = y + x
      | Z = z + atan(1/2^i) if z < 0, otherwise
      |    = z - atan(1/2^i)
  x : Inport
  y : Inport  Port=2
  z : Inport  Port=3
  MCode : xbsIndex_r4/MCode  mfname=cordic_pe_lat1  explicit_period=off  period=1  dbl_ovrd=off  enable_stdout=off  enable_debug=off  suppress_output=off  defparams={'shbits',ii,'epsilon', epsilon_k,'nbits', pe_nbits,'binpt', pe_binpt,'lat',pipeline}  hide_port_list={}  block_type=mcode
      settings: xl_area=[0, 0, 0, 0, 0, 0, 0]  block_version=8.1
  X : Outport
  Y : Outport  Port=2
  Z : Outport  Port=3
  wires:
  MCode/3 -> Z/1
  MCode/2 -> Y/1
  MCode/1 -> X/1
  z/1 -> MCode/3
  y/1 -> MCode/2
  x/1 -> MCode/1

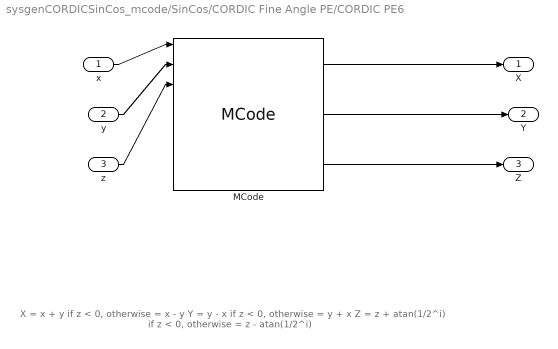
== system sysgenCORDICSinCos_mcode/SinCos/CORDIC Fine Angle PE/CORDIC PE6 ==
  note: X = x + y if z < 0, otherwise
      |    = x - y
      | Y = y - x if z < 0, otherwise
      |    = y + x
      | Z = z + atan(1/2^i) if z < 0, otherwise
      |    = z - atan(1/2^i)
  x : Inport
  y : Inport  Port=2
  z : Inport  Port=3
  MCode : xbsIndex_r4/MCode  mfname=cordic_pe_lat1  explicit_period=off  period=1  dbl_ovrd=off  enable_stdout=off  enable_debug=off  suppress_output=off  defparams={'shbits',ii,'epsilon', epsilon_k,'nbits', pe_nbits,'binpt', pe_binpt,'lat',pipeline}  hide_port_list={}  block_type=mcode
      settings: xl_area=[0, 0, 0, 0, 0, 0, 0]  block_version=8.1
  X : Outport
  Y : Outport  Port=2
  Z : Outport  Port=3
  wires:
  MCode/3 -> Z/1
  MCode/2 -> Y/1
  MCode/1 -> X/1
  z/1 -> MCode/3
  y/1 -> MCode/2
  x/1 -> MCode/1

== system sysgenCORDICSinCos_mcode/SinCos/CORDIC Fine Angle PE/CORDIC PE7 ==
  note: X = x + y if z < 0, otherwise
      |    = x - y
      | Y = y - x if z < 0, otherwise
      |    = y + x
      | Z = z + atan(1/2^i) if z < 0, otherwise
      |    = z - atan(1/2^i)
  x : Inport
  y : Inport  Port=2
  z : Inport  Port=3
  MCode : xbsIndex_r4/MCode  mfname=cordic_pe_lat1  explicit_period=off  period=1  dbl_ovrd=off  enable_stdout=off  enable_debug=off  suppress_output=off  defparams={'shbits',ii,'epsilon', epsilon_k,'nbits', pe_nbits,'binpt', pe_binpt,'lat',pipeline}  hide_port_list={}  block_type=mcode
      settings: xl_area=[0, 0, 0, 0, 0, 0, 0]  block_version=8.1
  X : Outport
  Y : Outport  Port=2
  Z : Outport  Port=3
  wires:
  MCode/3 -> Z/1
  MCode/2 -> Y/1
  MCode/1 -> X/1
  z/1 -> MCode/3
  y/1 -> MCode/2
  x/1 -> MCode/1

== system sysgenCORDICSinCos_mcode/SinCos/CORDIC Fine Angle PE/CORDIC PE8 ==
  note: X = x + y if z < 0, otherwise
      |    = x - y
      | Y = y - x if z < 0, otherwise
      |    = y + x
      | Z = z + atan(1/2^i) if z < 0, otherwise
      |    = z - atan(1/2^i)
  x : Inport
  y : Inport  Port=2
  z : Inport  Port=3
  MCode : xbsIndex_r4/MCode  mfname=cordic_pe_lat1  explicit_period=off  period=1  dbl_ovrd=off  enable_stdout=off  enable_debug=off  suppress_output=off  defparams={'shbits',ii,'epsilon', epsilon_k,'nbits', pe_nbits,'binpt', pe_binpt,'lat',pipeline}  hide_port_list={}  block_type=mcode
      settings: xl_area=[0, 0, 0, 0, 0, 0, 0]  block_version=8.1
  X : Outport
  Y : Outport  Port=2
  Z : Outport  Port=3
  wires:
  MCode/3 -> Z/1
  MCode/2 -> Y/1
  MCode/1 -> X/1
  z/1 -> MCode/3
  y/1 -> MCode/2
  x/1 -> MCode/1
